simulink model "NotchFilter"  (Simulink 8.9)
settings: Solver=VariableStepAuto  StartTime=0.0  StopTime=20.0  RelTol=1e-3
undefined symbols (not defined in the file): AP_PitchLoop_Notch1BWfactor, AP_PitchLoop_Notch1CosFreqNorm, Ts
settings Model: SuppressorTable=22 serialization::archive 11 0 6 0 0 0 0 0  Creator=hbolandhemmat  LastModifiedBy=hbolandhemmat
settings DataIOCC: LimitDataPoints=off  SaveFormat=Dataset  SignalLoggingSaveFormat=Dataset
settings OptimizationCC: LifeSpan=auto
settings DebuggingCC: UnderspecifiedInitializationDetection=Simplified  MergeDetectMultiDrivingBlocksExec=error  FcnCallInpInsideContextMsg=error  StateNameClashWarn=none  SFUnexpectedBacktrackingDiag=error  SFNoUnconditionalDefaultTransitionDiag=error  SFExecutionAtInitializationDiag=warning
settings HardwareCC: ProdBitPerPointer=64  ProdBitPerSizeT=64  ProdBitPerPtrDiffT=64  ProdLargestAtomicFloat=Float  ProdIntDivRoundTo=Zero  ProdEndianess=LittleEndian  ProdWordSize=64  ProdHWDeviceType=Intel->x86-64 (Windows64)
settings ModelReferenceCC: PropagateSignalLabelsOutOfModel=on
settings GRTTargetCC: TargetLangStandard=C99 (ISO)  GeneratePreprocessorConditionals=Use local settings  CombineOutputUpdateFcns=on  GRTInterface=off
settings ConfigComp: CovMetricSettings=dwe  CovHtmlReporting=off  CovSaveCumulativeToWorkspaceVar=off  CovSaveSingleToWorkspaceVar=off  CovExternalEMLEnable=on

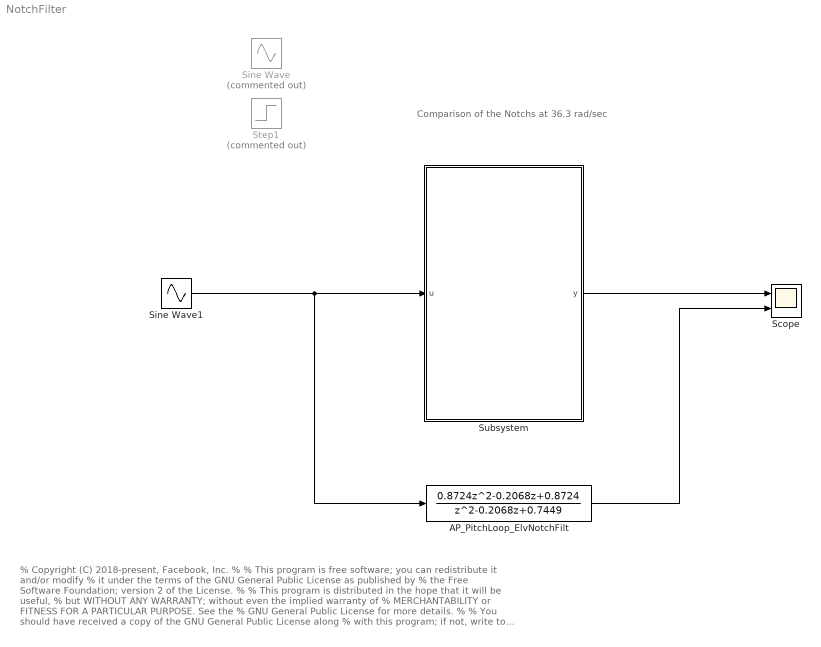
== system NotchFilter ==
  note: Comparison of the Notchs at 36.3 rad/sec
  note: % Copyright (C) 2018-present, Facebook, Inc.
      | %
      | % This program is free software; you can redistribute it and/or modify
      | % it under the terms of the GNU General Public License as published by
      | % the Free Software Foundation; version 2 of the License.
      | %
      | % This program is distributed in the hope that it will be useful,
      | % but WITHOUT ANY WARRANTY; without even the implied warranty of
      | % MERCHANTABILITY or FITNESS FOR A PARTICULAR PURPOSE. See the
      | % GNU General Public License for more details.
      | %
      | % You should have received a copy of the GNU General Public License along
      | % with this program; if not, write to the Free Software Foundation, Inc.,
      | % 51 Franklin Street, Fifth Floor, Boston, MA 02110-1301 USA.
  AP_PitchLoop_ElvNotchFilt : DiscreteTransferFcn  Numerator=[0.8724 -0.2068 0.8724]  Denominator=[1 -0.2068 0.7449]  SampleTime=Ts
  Scope : Scope  NumInputPorts=2
  Sine Wave : Sin  Commented=on  Frequency=36.3  SampleTime=Ts
  Sine Wave1 : Sin  Frequency=36  SampleTime=Ts
  Step1 : Step  Commented=on  SampleTime=0
  Subsystem : Subsystem
  wires:
  Sine Wave1/1 -> Subsystem/1(u), AP_PitchLoop_ElvNotchFilt/1
  Subsystem/1(y) -> Scope/1
  AP_PitchLoop_ElvNotchFilt/1 -> Scope/2

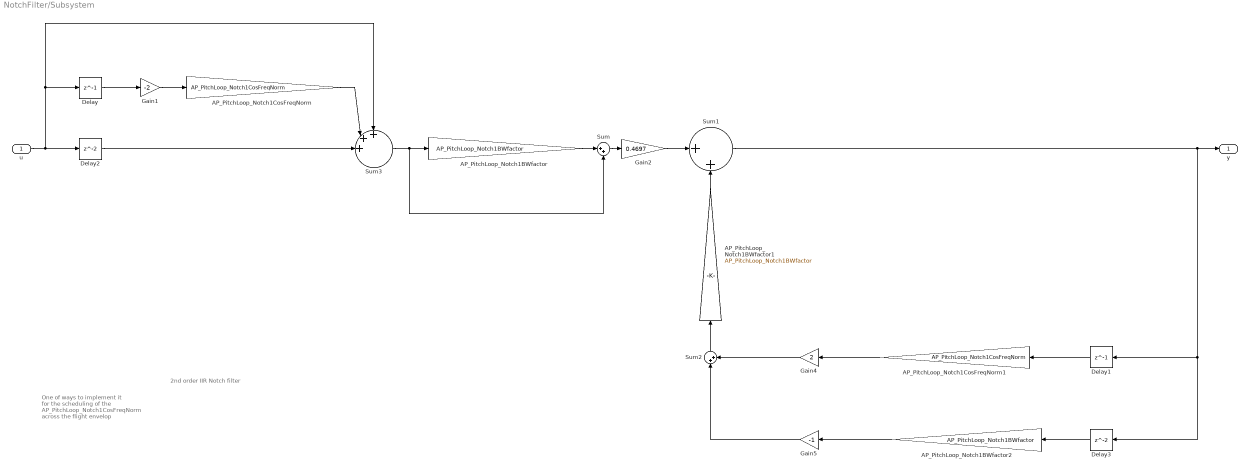
== system NotchFilter/Subsystem ==
  note: One of ways to implement it for the scheduling of the AP_PitchLoop_Notch1CosFreqNorm across the flight envelop
  note: 2nd order IIR Notch filter
  u : Inport
  AP_PitchLoop_Notch1BWfactor : Gain  Gain=AP_PitchLoop_Notch1BWfactor
  AP_PitchLoop_Notch1BWfactor1 : Gain  Gain=AP_PitchLoop_Notch1BWfactor
  AP_PitchLoop_Notch1BWfactor2 : Gain  Gain=AP_PitchLoop_Notch1BWfactor
  AP_PitchLoop_Notch1CosFreqNorm : Gain  Gain=AP_PitchLoop_Notch1CosFreqNorm
  AP_PitchLoop_Notch1CosFreqNorm1 : Gain  Gain=AP_PitchLoop_Notch1CosFreqNorm
  Delay : Delay  DelayLength=1  InitialCondition=0  SampleTime=Ts
  Delay1 : Delay  DelayLength=1  InitialCondition=0  SampleTime=Ts
  Delay2 : Delay  InitialCondition=0  SampleTime=Ts
  Delay3 : Delay  InitialCondition=0  SampleTime=Ts
  Gain1 : Gain  Gain=-2
  Gain2 : Gain  Gain=0.4697
  Gain4 : Gain  Gain=2
  Gain5 : Gain  Gain=-1
  Sum : Sum  Inputs=|++
  Sum1 : Sum  Inputs=|++
  Sum2 : Sum  Inputs=|++
  Sum3 : Sum  Inputs=+++||
  y : Outport
  wires:
  Sum/1 -> Gain2/1
  AP_PitchLoop_Notch1BWfactor/1 -> Sum/1
  AP_PitchLoop_Notch1CosFreqNorm/1 -> Sum3/2
  u/1 -> Delay/1, Sum3/1, Delay2/1
  Sum1/1 -> y/1, Delay1/1, Delay3/1
  AP_PitchLoop_Notch1BWfactor2/1 -> Gain5/1
  Delay3/1 -> AP_PitchLoop_Notch1BWfactor2/1
  Gain1/1 -> AP_PitchLoop_Notch1CosFreqNorm/1
  Delay1/1 -> AP_PitchLoop_Notch1CosFreqNorm1/1
  Delay2/1 -> Sum3/3
  Delay/1 -> Gain1/1
  AP_PitchLoop_Notch1CosFreqNorm1/1 -> Gain4/1
  Sum3/1 -> Sum/2, AP_PitchLoop_Notch1BWfactor/1
  Gain2/1 -> Sum1/1
  Gain4/1 -> Sum2/2
  Gain5/1 -> Sum2/1
  AP_PitchLoop_Notch1BWfactor1/1 -> Sum1/2
  Sum2/1 -> AP_PitchLoop_Notch1BWfactor1/1
